simulink model "TOAD_1DOF_model"  (R2023b)
settings: Solver=VariableStepAuto  StartTime=reference_trajectory(1, 1)  StopTime=reference_trajectory(end, 1)  RelTol=1e-12  AbsTol=1e-12
model workspace (MAT data in the model file):
  K = [1 0 0]
  m_inert = 136.0776
  m_propellant = 272.1552
  reference_trajectory = [0 0.0600600600601 0.12012012012 0.18018018018 0.24024024024 0.3003003003 0.36036036036 0.42042042042 0.48048048048 0.540540540541 0.600600600601 0.660660660661 ... (2000 elements, 1000x2)]
libraries: dspsigops x1
settings Model: Creator=anigo  LastModifiedBy=anigo
settings DataIOCC: SaveFormat=Array  SignalLogging=off  DSMLogging=off  ReturnWorkspaceOutputs=off

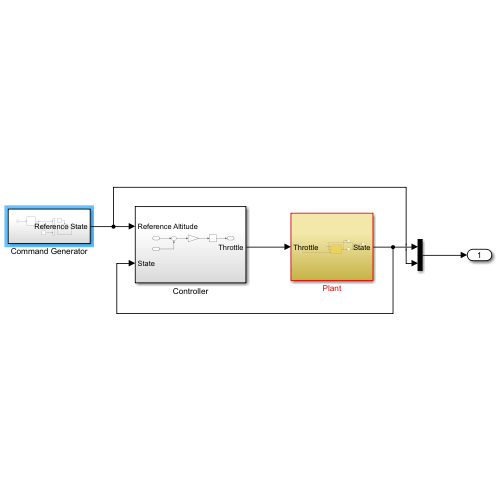
[thumbnail: Simulink's stored preview of the top-level diagram]
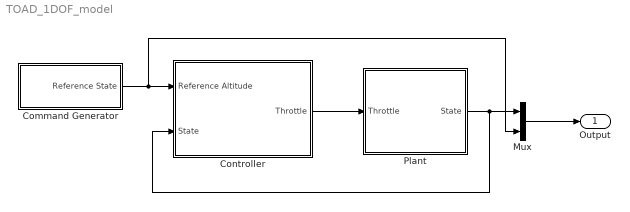
== system TOAD_1DOF_model ==
  Command Generator : Subsystem
  Controller : Subsystem
  Mux : Mux  Inputs=2
  Plant : Subsystem
  Output : Outport
  wires:
  Command Generator/1(Reference State) -> Mux/2, Controller/1(Reference Altitude)
  Controller/1(Throttle) -> Plant/1(Throttle)
  Plant/1(State) -> Mux/1, Controller/2(State)
  Mux/1 -> Output/1

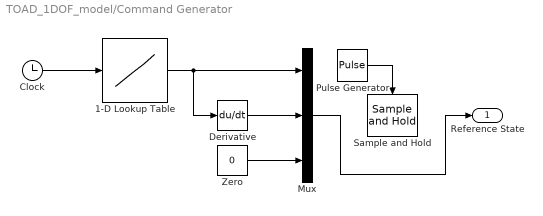
== system TOAD_1DOF_model/Command Generator ==
  1-D Lookup Table : Lookup_n-D  NumberOfTableDimensions=1  BreakpointsForDimension1=reference_trajectory(:, 1)  Table=reference_trajectory(:, 2)  InternalRulePriority=Speed  RndMeth=Simplest
  Clock : Clock
  Derivative : Derivative
  Mux : Mux  Inputs=3
  Pulse Generator : DiscretePulseGenerator  PulseType=Time based  Period=1/100  PulseWidth=5
  Sample and Hold : dspsigops/Sample and Hold  trig=Rising edge  initCond=0  latchinput=off
  Zero : Constant  Value=0  OutDataTypeStr=Inherit: Inherit via back propagation
  Reference State : Outport
  wires:
  Clock/1 -> 1-D Lookup Table/1
  1-D Lookup Table/1 -> Mux/1, Derivative/1
  Derivative/1 -> Mux/2
  Zero/1 -> Mux/3
  Pulse Generator/1 -> Sample and Hold/Trigger
  Mux/1 -> Reference State/1

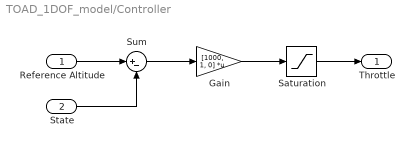
== system TOAD_1DOF_model/Controller ==
  Reference Altitude : Inport
  State : Inport  Port=2
  Gain : Gain  Gain=[1000, 1, 0]  Multiplication=Matrix(K*u)
  Saturation : Saturate  UpperLimit=100  LowerLimit=40  ZeroCross=off
  Sum : Sum  Inputs=|+-
  Throttle : Outport
  wires:
  Reference Altitude/1 -> Sum/1
  State/1 -> Sum/2
  Sum/1 -> Gain/1
  Gain/1 -> Saturation/1
  Saturation/1 -> Throttle/1

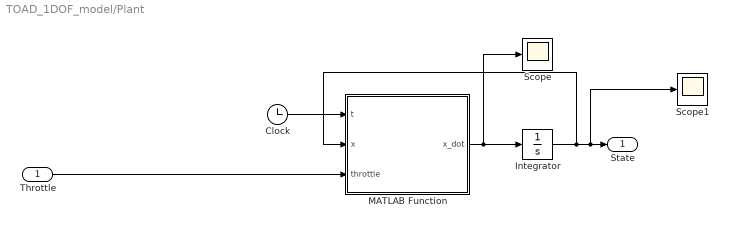
== system TOAD_1DOF_model/Plant ==
  Throttle : Inport
  Clock : Clock
  Integrator : Integrator  InitialCondition=[reference_trajectory(1, 2); 0; m_inert + m_propellant]
  MATLAB Function : MATLAB Function  TreatAsAtomicUnit=on
  Scope : Scope
  Scope1 : Scope
  State : Outport
  wires:
  Throttle/1 -> MATLAB Function/3(throttle)
  Integrator/1 -> Scope1/1, State/1, MATLAB Function/2(x)
  Clock/1 -> MATLAB Function/1(t)
  MATLAB Function/1(x_dot) -> Scope/1, Integrator/1

== matlab function TOAD_1DOF_model/Plant/MATLAB Function ==
  data: t input; x_dot output; x input; throttle input; m_inert parameter
function x_dot = fcn(t, x, throttle, m_inert)
    coder.extrinsic('./lib/EOMS.m');
    x_dot = EOMS(t, x, throttle, m_inert);
end
